simulink model "PRO_TestHarness"  (Simulink 8.6)
settings: Solver=ode45  StartTime=0.0  StopTime=10.0  RelTol=1e-3
PreLoadFcn:
  | addpath('./Workspace/')
  | load('./Workspace/EnvVar.mat')
  | if exist('tl_preloadfcn','file'), tl_preloadfcn(gcs,402); end
PostLoadFcn:
  | if exist('tl_postloadfcn','file'), tl_postloadfcn(gcs,402); end
InitFcn:
  | if exist('tlds_init','file'), tlds_init(gcs); end
StartFcn:
  | if exist('tlds_start','file'), tlds_start(gcs); end
StopFcn:
  | if exist('tlds_stop','file'), tlds_stop(gcs); end
undefined symbols (not defined in the file or in its folder): ddv, sigbuilder_block, Ts
libraries: tllib x19, simulink x2
(part 2 of 5)

== system PRO_TestHarness/PRO_AC_ProductionCycles/Subsystem/PRO_AC_ProductionCycles/PRO_AC_ProductionCycles/PRO_runProductionCycles ==
  u8RequestedCycle : Inport  OutDataTypeStr=uint8  PortDimensions=1  mask(TL_Inport){data={'autosar',{'useautosarcommunication',1,'kind',4,'senderreceiverport','prrDiagRequestCycle','dataelement','u8RequestedCycle','interrunnablevariable','BPA_AC_BeltParkingAlgorithm/IRV/u8BeltParkingAuthorizationState','clientserverport','pclDiagRequestCycle','operation','GetDiagRequestCycle'},'date',736040.52059280092}}
      settings: CopyFcn=if exist('tl_reset_reviewflag','file')==2,tl_reset_reviewflag(gcbh);end  DeleteFcn=if exist('delete_tlblock','file')==2,delete_tlblock(gcbh);end  NameChangeFcn=if exist('rename_tlblock','file')==2,rename_tlblock(gcbh);end  OpenFcn=if exist('tl_open_blockdlg','file')==2,tl_open_blockdlg(gcbh);else,open_system(gcbh,'parameter');end
      mask Help: eval(['if exist(''tl_online_help'',''file'') == 2, tl_online_help(''Topic'',''TL_Inport''),else, web([''jar:file:///'',matlabroot,''/help/toolbox/simulink/help.jar!/slref/' lower(get_param(gcbh,'Blocktype')) '.html''], ''-helpbrowser''),end'])
      mask Display: plot([0.2 0.35 NaN 0.65 0.8],[0 1 NaN 0 1]);
  u8ExecutedCycle : Inport  Port=2  PortDimensions=1  mask(TL_Inport){data={'autosar',{'useautosarcommunication',1,'senderreceiverport','prrExecutedCycle','dataelement','u8CycleNumber'},'date',735609.60262215277}}
      settings: CopyFcn=if exist('tl_reset_reviewflag','file')==2,tl_reset_reviewflag(gcbh);end  DeleteFcn=if exist('delete_tlblock','file')==2,delete_tlblock(gcbh);end  NameChangeFcn=if exist('rename_tlblock','file')==2,rename_tlblock(gcbh);end  OpenFcn=if exist('tl_open_blockdlg','file')==2,tl_open_blockdlg(gcbh);else,open_system(gcbh,'parameter');end
      mask Help: eval(['if exist(''tl_online_help'',''file'') == 2, tl_online_help(''Topic'',''TL_Inport''),else, web([''jar:file:///'',matlabroot,''/help/toolbox/simulink/help.jar!/slref/' lower(get_param(gcbh,'Blocktype')) '.html''], ''-helpbrowser''),end'])
      mask Display: plot([0.2 0.35 NaN 0.65 0.8],[0 1 NaN 0 1]);
  Trigger : TriggerPort  RequirementInfo={} %GIDa_248c7611_0acb_4b44_ba04_7ddf45d8e22c  TriggerType=function-call
  Constant2 : Constant  Value=ddv('BFD/CFG_K_MASK_PRO_DTC_ABORTION_CONTEXT')  OutDataTypeStr=uint8  mask(TL_Constant){data={'output',{'variable','BFD/CFG_K_MASK_PRO_DTC_ABORTION_CONTEXT'},'date',735893.56781245372}}
      settings: DeleteFcn=if exist('delete_tlblock','file')==2,delete_tlblock(gcbh);end  NameChangeFcn=if exist('rename_tlblock','file')==2,rename_tlblock(gcbh);end  OpenFcn=if exist('tl_open_blockdlg','file')==2,tl_open_blockdlg(gcbh);else,open_system(gcbh,'parameter');end
      mask Help: eval(['if exist(''tl_online_help'',''file'') == 2, tl_online_help(''Topic'',''TL_Constant''),else, web([''jar:file:///'',matlabroot,''/help/toolbox/simulink/help.jar!/slref/' lower(get_param(gcbh,'Blocktype')) '.html''], ''-helpbrowser''),end'])
      mask Display: plot([-0.05, 1.05, NaN, -0.05, 1.05],[.01, .01, NaN, .99, .99])
  Constant4 : Constant  Value=ddv('BFD/CFG_K_MASK_PRO_DTC_INHIBITION_CONTEXT')  OutDataTypeStr=uint8  mask(TL_Constant){data={'output',{'variable','BFD/CFG_K_MASK_PRO_DTC_INHIBITION_CONTEXT'},'date',735893.56753854163}}
      settings: DeleteFcn=if exist('delete_tlblock','file')==2,delete_tlblock(gcbh);end  NameChangeFcn=if exist('rename_tlblock','file')==2,rename_tlblock(gcbh);end  OpenFcn=if exist('tl_open_blockdlg','file')==2,tl_open_blockdlg(gcbh);else,open_system(gcbh,'parameter');end
      mask Help: eval(['if exist(''tl_online_help'',''file'') == 2, tl_online_help(''Topic'',''TL_Constant''),else, web([''jar:file:///'',matlabroot,''/help/toolbox/simulink/help.jar!/slref/' lower(get_param(gcbh,'Blocktype')) '.html''], ''-helpbrowser''),end'])
      mask Display: plot([-0.05, 1.05, NaN, -0.05, 1.05],[.01, .01, NaN, .99, .99])
  Dem_GetEventStatus : Subsystem  RequirementInfo={} %GIDa_e11a4632_883c_4bf9_94c9_e29d5c312dd8  TreatAsAtomicUnit=on
  Dem_GetEventStatus1 : Subsystem  RequirementInfo={} %GIDa_4470c0a2_043c_4322_94f3_9034f61d5407  TreatAsAtomicUnit=on
  Flags_PRO1 : Subsystem
  Flags_PRO2 : Subsystem
  PRO enabled : Subsystem  TreatAsAtomicUnit=on
  Runnable : tllib/Function  data={'autosar',{'useautosarspecification',1,'softwarecomponent','AUTOLIV/SoftwareComponents/PRO/PRO_AC_ProductionCycles','runnable','PRO_runProductionCycles'},'date',736811.32660734956}  displayString=RUNNABLE
  SCA_runCheckSystemContext1 : Subsystem  RequirementInfo={} %GIDa_959a77de_17ea_490b_b4e4_7bbcc1f3502a  TreatAsAtomicUnit=on
  SCA_runCheckSystemContext2 : Subsystem  RequirementInfo={} %GIDa_6e6b4e65_c2e0_44f1_91eb_aa27d502d2da  TreatAsAtomicUnit=on
  b8TriggeringOrder_PRO1 : Outport  PortDimensions=1  mask(TL_Outport){data={'autosar',{'useautosarcommunication',1,'senderreceiverport','psrAlgo_Flags_PRO1','dataelement','b8TriggerFlag'},'date',735664.44418690971}}
      settings: CopyFcn=if exist('tl_reset_reviewflag','file')==2,tl_reset_reviewflag(gcbh);end  DeleteFcn=if exist('delete_tlblock','file')==2,delete_tlblock(gcbh);end  NameChangeFcn=if exist('rename_tlblock','file')==2,rename_tlblock(gcbh);end  OpenFcn=if exist('tl_open_blockdlg','file')==2,tl_open_blockdlg(gcbh);else,open_system(gcbh,'parameter');end
      mask Help: eval(['if exist(''tl_online_help'',''file'') == 2, tl_online_help(''Topic'',''TL_Outport''),else, web([''jar:file:///'',matlabroot,''/help/toolbox/simulink/help.jar!/slref/' lower(get_param(gcbh,'Blocktype')) '.html''], ''-helpbrowser''),end'])
      mask Display: plot([0.2 0.35 NaN 0.65 0.8],[0 1 NaN 0 1]);
  b8AbortionOrder_PRO1 : Outport  Port=2  PortDimensions=1  mask(TL_Outport){data={'autosar',{'useautosarcommunication',1,'senderreceiverport','psrAlgo_Flags_PRO1','dataelement','b8InterruptFlag'},'date',735664.44679810188}}
      settings: CopyFcn=if exist('tl_reset_reviewflag','file')==2,tl_reset_reviewflag(gcbh);end  DeleteFcn=if exist('delete_tlblock','file')==2,delete_tlblock(gcbh);end  NameChangeFcn=if exist('rename_tlblock','file')==2,rename_tlblock(gcbh);end  OpenFcn=if exist('tl_open_blockdlg','file')==2,tl_open_blockdlg(gcbh);else,open_system(gcbh,'parameter');end
      mask Help: eval(['if exist(''tl_online_help'',''file'') == 2, tl_online_help(''Topic'',''TL_Outport''),else, web([''jar:file:///'',matlabroot,''/help/toolbox/simulink/help.jar!/slref/' lower(get_param(gcbh,'Blocktype')) '.html''], ''-helpbrowser''),end'])
      mask Display: plot([0.2 0.35 NaN 0.65 0.8],[0 1 NaN 0 1]);
  b8PreActivationFlag_PRO1 : Outport  Port=3  PortDimensions=1  mask(TL_Outport){data={'autosar',{'useautosarcommunication',1,'senderreceiverport','psrAlgo_Flags_PRO1','dataelement','b8PreActivationFlag'},'date',735664.44689250004}}
      settings: CopyFcn=if exist('tl_reset_reviewflag','file')==2,tl_reset_reviewflag(gcbh);end  DeleteFcn=if exist('delete_tlblock','file')==2,delete_tlblock(gcbh);end  NameChangeFcn=if exist('rename_tlblock','file')==2,rename_tlblock(gcbh);end  OpenFcn=if exist('tl_open_blockdlg','file')==2,tl_open_blockdlg(gcbh);else,open_system(gcbh,'parameter');end
      mask Help: eval(['if exist(''tl_online_help'',''file'') == 2, tl_online_help(''Topic'',''TL_Outport''),else, web([''jar:file:///'',matlabroot,''/help/toolbox/simulink/help.jar!/slref/' lower(get_param(gcbh,'Blocktype')) '.html''], ''-helpbrowser''),end'])
      mask Display: plot([0.2 0.35 NaN 0.65 0.8],[0 1 NaN 0 1]);
  b8PreConditionsFlag_PRO1 : Outport  Port=4  PortDimensions=1  mask(TL_Outport){data={'autosar',{'useautosarcommunication',1,'senderreceiverport','psrAlgo_Flags_PRO1','dataelement','b8PreConditionsFlag'},'date',735664.44697152777}}
      settings: CopyFcn=if exist('tl_reset_reviewflag','file')==2,tl_reset_reviewflag(gcbh);end  DeleteFcn=if exist('delete_tlblock','file')==2,delete_tlblock(gcbh);end  NameChangeFcn=if exist('rename_tlblock','file')==2,rename_tlblock(gcbh);end  OpenFcn=if exist('tl_open_blockdlg','file')==2,tl_open_blockdlg(gcbh);else,open_system(gcbh,'parameter');end
      mask Help: eval(['if exist(''tl_online_help'',''file'') == 2, tl_online_help(''Topic'',''TL_Outport''),else, web([''jar:file:///'',matlabroot,''/help/toolbox/simulink/help.jar!/slref/' lower(get_param(gcbh,'Blocktype')) '.html''], ''-helpbrowser''),end'])
      mask Display: plot([0.2 0.35 NaN 0.65 0.8],[0 1 NaN 0 1]);
  u8TriggeringSource_PRO1 : Outport  Port=5  PortDimensions=1  mask(TL_Outport){data={'autosar',{'useautosarcommunication',1,'senderreceiverport','psrAlgo_Flags_PRO1','dataelement','u8TriggeringSource'},'date',735664.44705670141}}
      settings: CopyFcn=if exist('tl_reset_reviewflag','file')==2,tl_reset_reviewflag(gcbh);end  DeleteFcn=if exist('delete_tlblock','file')==2,delete_tlblock(gcbh);end  NameChangeFcn=if exist('rename_tlblock','file')==2,rename_tlblock(gcbh);end  OpenFcn=if exist('tl_open_blockdlg','file')==2,tl_open_blockdlg(gcbh);else,open_system(gcbh,'parameter');end
      mask Help: eval(['if exist(''tl_online_help'',''file'') == 2, tl_online_help(''Topic'',''TL_Outport''),else, web([''jar:file:///'',matlabroot,''/help/toolbox/simulink/help.jar!/slref/' lower(get_param(gcbh,'Blocktype')) '.html''], ''-helpbrowser''),end'])
      mask Display: plot([0.2 0.35 NaN 0.65 0.8],[0 1 NaN 0 1]);
  b8TriggeringOrder_PRO2 : Outport  Port=6  PortDimensions=1  mask(TL_Outport){data={'autosar',{'useautosarcommunication',1,'senderreceiverport','psrAlgo_Flags_PRO2','dataelement','b8TriggerFlag'},'date',735664.44714405097}}
      settings: CopyFcn=if exist('tl_reset_reviewflag','file')==2,tl_reset_reviewflag(gcbh);end  DeleteFcn=if exist('delete_tlblock','file')==2,delete_tlblock(gcbh);end  NameChangeFcn=if exist('rename_tlblock','file')==2,rename_tlblock(gcbh);end  OpenFcn=if exist('tl_open_blockdlg','file')==2,tl_open_blockdlg(gcbh);else,open_system(gcbh,'parameter');end
      mask Help: eval(['if exist(''tl_online_help'',''file'') == 2, tl_online_help(''Topic'',''TL_Outport''),else, web([''jar:file:///'',matlabroot,''/help/toolbox/simulink/help.jar!/slref/' lower(get_param(gcbh,'Blocktype')) '.html''], ''-helpbrowser''),end'])
      mask Display: plot([0.2 0.35 NaN 0.65 0.8],[0 1 NaN 0 1]);
  b8AbortionOrder_PRO2 : Outport  Port=7  PortDimensions=1  mask(TL_Outport){data={'autosar',{'useautosarcommunication',1,'senderreceiverport','psrAlgo_Flags_PRO2','dataelement','b8InterruptFlag'},'date',735664.44722253468}}
      settings: CopyFcn=if exist('tl_reset_reviewflag','file')==2,tl_reset_reviewflag(gcbh);end  DeleteFcn=if exist('delete_tlblock','file')==2,delete_tlblock(gcbh);end  NameChangeFcn=if exist('rename_tlblock','file')==2,rename_tlblock(gcbh);end  OpenFcn=if exist('tl_open_blockdlg','file')==2,tl_open_blockdlg(gcbh);else,open_system(gcbh,'parameter');end
      mask Help: eval(['if exist(''tl_online_help'',''file'') == 2, tl_online_help(''Topic'',''TL_Outport''),else, web([''jar:file:///'',matlabroot,''/help/toolbox/simulink/help.jar!/slref/' lower(get_param(gcbh,'Blocktype')) '.html''], ''-helpbrowser''),end'])
      mask Display: plot([0.2 0.35 NaN 0.65 0.8],[0 1 NaN 0 1]);
  b8PreActivationFlag_PRO2 : Outport  Port=8  PortDimensions=1  mask(TL_Outport){data={'autosar',{'useautosarcommunication',1,'senderreceiverport','psrAlgo_Flags_PRO2','dataelement','b8PreActivationFlag'},'date',735664.44730300922}}
      settings: CopyFcn=if exist('tl_reset_reviewflag','file')==2,tl_reset_reviewflag(gcbh);end  DeleteFcn=if exist('delete_tlblock','file')==2,delete_tlblock(gcbh);end  NameChangeFcn=if exist('rename_tlblock','file')==2,rename_tlblock(gcbh);end  OpenFcn=if exist('tl_open_blockdlg','file')==2,tl_open_blockdlg(gcbh);else,open_system(gcbh,'parameter');end
      mask Help: eval(['if exist(''tl_online_help'',''file'') == 2, tl_online_help(''Topic'',''TL_Outport''),else, web([''jar:file:///'',matlabroot,''/help/toolbox/simulink/help.jar!/slref/' lower(get_param(gcbh,'Blocktype')) '.html''], ''-helpbrowser''),end'])
      mask Display: plot([0.2 0.35 NaN 0.65 0.8],[0 1 NaN 0 1]);
  b8PreConditionsFlag_PRO2 : Outport  Port=9  PortDimensions=1  mask(TL_Outport){data={'autosar',{'useautosarcommunication',1,'senderreceiverport','psrAlgo_Flags_PRO2','dataelement','b8PreConditionsFlag'},'date',735664.44739415508}}
      settings: CopyFcn=if exist('tl_reset_reviewflag','file')==2,tl_reset_reviewflag(gcbh);end  DeleteFcn=if exist('delete_tlblock','file')==2,delete_tlblock(gcbh);end  NameChangeFcn=if exist('rename_tlblock','file')==2,rename_tlblock(gcbh);end  OpenFcn=if exist('tl_open_blockdlg','file')==2,tl_open_blockdlg(gcbh);else,open_system(gcbh,'parameter');end
      mask Help: eval(['if exist(''tl_online_help'',''file'') == 2, tl_online_help(''Topic'',''TL_Outport''),else, web([''jar:file:///'',matlabroot,''/help/toolbox/simulink/help.jar!/slref/' lower(get_param(gcbh,'Blocktype')) '.html''], ''-helpbrowser''),end'])
      mask Display: plot([0.2 0.35 NaN 0.65 0.8],[0 1 NaN 0 1]);
  u8TriggeringSource_PRO2 : Outport  Port=10  PortDimensions=1  mask(TL_Outport){data={'autosar',{'useautosarcommunication',1,'senderreceiverport','psrAlgo_Flags_PRO2','dataelement','u8TriggeringSource'},'date',735664.44747879624}}
      settings: CopyFcn=if exist('tl_reset_reviewflag','file')==2,tl_reset_reviewflag(gcbh);end  DeleteFcn=if exist('delete_tlblock','file')==2,delete_tlblock(gcbh);end  NameChangeFcn=if exist('rename_tlblock','file')==2,rename_tlblock(gcbh);end  OpenFcn=if exist('tl_open_blockdlg','file')==2,tl_open_blockdlg(gcbh);else,open_system(gcbh,'parameter');end
      mask Help: eval(['if exist(''tl_online_help'',''file'') == 2, tl_online_help(''Topic'',''TL_Outport''),else, web([''jar:file:///'',matlabroot,''/help/toolbox/simulink/help.jar!/slref/' lower(get_param(gcbh,'Blocktype')) '.html''], ''-helpbrowser''),end'])
      mask Display: plot([0.2 0.35 NaN 0.65 0.8],[0 1 NaN 0 1]);
  wires:
  u8ExecutedCycle/1 -> PRO enabled/2(u8ExecutedCycle)
  SCA_runCheckSystemContext1/1(b8SystemContext) -> PRO enabled/3(b8SystemContextInhibition)
  SCA_runCheckSystemContext2/1(b8SystemContext) -> PRO enabled/4(b8SystemContextAbortion)
  Constant2/1 -> SCA_runCheckSystemContext2/1(u16SystemContextsToCheck)
  u8RequestedCycle/1 -> PRO enabled/1(u8RequestedCycle)
  Constant4/1 -> SCA_runCheckSystemContext1/1(u16SystemContextsToCheck)
  PRO enabled/1(psrAlgoFlags_PRO1) -> Flags_PRO1/1(In1)
  Flags_PRO1/1(Out1) -> b8TriggeringOrder_PRO1/1
  Flags_PRO1/2(Out2) -> b8AbortionOrder_PRO1/1
  Flags_PRO1/3(Out3) -> b8PreActivationFlag_PRO1/1
  Flags_PRO1/4(Out4) -> b8PreConditionsFlag_PRO1/1
  Flags_PRO1/5(Out5) -> u8TriggeringSource_PRO1/1
  Flags_PRO2/1(Out1) -> b8TriggeringOrder_PRO2/1
  Flags_PRO2/2(Out2) -> b8AbortionOrder_PRO2/1
  Flags_PRO2/3(Out3) -> b8PreActivationFlag_PRO2/1
  Flags_PRO2/4(Out4) -> b8PreConditionsFlag_PRO2/1
  Flags_PRO2/5(Out5) -> u8TriggeringSource_PRO2/1
  PRO enabled/2(psrAlgoFlags_PRO2) -> Flags_PRO2/1(In1)
  Dem_GetEventStatus1/1(u8EventStatus) -> PRO enabled/5(u8UVDuringTensioningEventStatus)
  Dem_GetEventStatus/1(u8EventStatus) -> PRO enabled/6(u8OverVoltageEventStatus)

== system PRO_TestHarness/PRO_AC_ProductionCycles/Subsystem/PRO_AC_ProductionCycles/PRO_AC_ProductionCycles/WriteSystemContextOutputs ==
  b8CyclesInhibitedByDTC1 : Inport
  b8CyclesAbortedByDTC : Inport  Port=2
  u8AecStatus_UVDuringTens1 : Inport  Port=3
  u8Status_OVO : Inport  Port=4
  Trigger : TriggerPort  RequirementInfo={} %GIDa_0b5c07fd_5561_4776_a0f4_36f279c5ca10  TriggerType=function-call
  Data Store Write1 : DataStoreWrite  DataStoreName=b8CyclesInhibitedByDTC  mask(TL_DataStoreWrite){data={'date',735893.56874431716}}
      settings: DeleteFcn=if exist('delete_tlblock','file')==2,delete_tlblock(gcbh);end  NameChangeFcn=if exist('rename_tlblock','file')==2,rename_tlblock(gcbh);end  OpenFcn=if exist('tl_open_blockdlg','file')==2,tl_open_blockdlg(gcbh);else,open_system(gcbh,'parameter');end
      mask Help: eval(['if exist(''tl_online_help'',''file'') == 2, tl_online_help(''Topic'',''TL_DataStoreWrite''),else, web([''jar:file:///'',matlabroot,''/help/toolbox/simulink/help.jar!/slref/' lower(get_param(gcbh,'Blocktype')) '.html''], ''-helpbrowser''),end'])
      mask Display: plot([-0.05, 1.05, NaN, -0.05, 1.05],[.01, .01, NaN, .99, .99])
  Data Store Write2 : DataStoreWrite  DataStoreName=b8CyclesAbortedByDTC  mask(TL_DataStoreWrite){data={'date',735893.56880297454}}
      settings: DeleteFcn=if exist('delete_tlblock','file')==2,delete_tlblock(gcbh);end  NameChangeFcn=if exist('rename_tlblock','file')==2,rename_tlblock(gcbh);end  OpenFcn=if exist('tl_open_blockdlg','file')==2,tl_open_blockdlg(gcbh);else,open_system(gcbh,'parameter');end
      mask Help: eval(['if exist(''tl_online_help'',''file'') == 2, tl_online_help(''Topic'',''TL_DataStoreWrite''),else, web([''jar:file:///'',matlabroot,''/help/toolbox/simulink/help.jar!/slref/' lower(get_param(gcbh,'Blocktype')) '.html''], ''-helpbrowser''),end'])
      mask Display: plot([-0.05, 1.05, NaN, -0.05, 1.05],[.01, .01, NaN, .99, .99])
  Data Store Write4 : DataStoreWrite  DataStoreName=u8Status_UVT  mask(TL_DataStoreWrite){data={'date',736231.39905967598}}
      settings: DeleteFcn=if exist('delete_tlblock','file')==2,delete_tlblock(gcbh);end  NameChangeFcn=if exist('rename_tlblock','file')==2,rename_tlblock(gcbh);end  OpenFcn=if exist('tl_open_blockdlg','file')==2,tl_open_blockdlg(gcbh);else,open_system(gcbh,'parameter');end
      mask Help: eval(['if exist(''tl_online_help'',''file'') == 2, tl_online_help(''Topic'',''TL_DataStoreWrite''),else, web([''jar:file:///'',matlabroot,''/help/toolbox/simulink/help.jar!/slref/' lower(get_param(gcbh,'Blocktype')) '.html''], ''-helpbrowser''),end'])
      mask Display: plot([-0.05, 1.05, NaN, -0.05, 1.05],[.01, .01, NaN, .99, .99])
  Data Store Write5 : DataStoreWrite  DataStoreName=u8Status_OVO  mask(TL_DataStoreWrite){data={'date',735987.71420101856}}
      settings: DeleteFcn=if exist('delete_tlblock','file')==2,delete_tlblock(gcbh);end  NameChangeFcn=if exist('rename_tlblock','file')==2,rename_tlblock(gcbh);end  OpenFcn=if exist('tl_open_blockdlg','file')==2,tl_open_blockdlg(gcbh);else,open_system(gcbh,'parameter');end
      mask Help: eval(['if exist(''tl_online_help'',''file'') == 2, tl_online_help(''Topic'',''TL_DataStoreWrite''),else, web([''jar:file:///'',matlabroot,''/help/toolbox/simulink/help.jar!/slref/' lower(get_param(gcbh,'Blocktype')) '.html''], ''-helpbrowser''),end'])
      mask Display: plot([-0.05, 1.05, NaN, -0.05, 1.05],[.01, .01, NaN, .99, .99])
  wires:
  b8CyclesInhibitedByDTC1/1 -> Data Store Write1/1
  b8CyclesAbortedByDTC/1 -> Data Store Write2/1
  u8AecStatus_UVDuringTens1/1 -> Data Store Write4/1
  u8Status_OVO/1 -> Data Store Write5/1

== system PRO_TestHarness/PRO_AC_ProductionCycles/Subsystem/PRO_AC_ProductionCycles/PRO_AC_ProductionCycles/PRO_runProductionCycles/Dem_GetEventStatus ==
  Data Store Read1 : DataStoreRead  DataStoreName=u8Status_OVO  mask(TL_DataStoreRead){data={'date',735987.66306642361}}
      settings: DeleteFcn=if exist('delete_tlblock','file')==2,delete_tlblock(gcbh);end  NameChangeFcn=if exist('rename_tlblock','file')==2,rename_tlblock(gcbh);end  OpenFcn=if exist('tl_open_blockdlg','file')==2,tl_open_blockdlg(gcbh);else,open_system(gcbh,'parameter');end
      mask Help: eval(['if exist(''tl_online_help'',''file'') == 2, tl_online_help(''Topic'',''TL_DataStoreRead''),else, web([''jar:file:///'',matlabroot,''/help/toolbox/simulink/help.jar!/slref/' lower(get_param(gcbh,'Blocktype')) '.html''], ''-helpbrowser''),end'])
      mask Display: plot([-0.05, 1.05, NaN, -0.05, 1.05],[.01, .01, NaN, .99, .99])
  Function1 : tllib/Function  RequirementInfo={} %GIDa_c22adf50_ccfc_4787_ab66_0286f94d3b05  data={'stepfunctionname','Rte_Call_pclSystemContext_CheckSystemContext','stepfunctionclass','EXTERN_FCN_SCA','functionarglist',{'u16SystemContextsToCheck';'b8SystemContextStatus_DTCInhibition'},'autosar',{'useautosarspecification',1,'functionrole',3,'clientport','pclEvtInfoBatPwrOverVoltage','operation','GetEventStatus','isimplementationforsilpil',0,'clientsoftwarecomponent','AUTOLIV/SoftwareComponents/PRO/PRO_AC_ProductionCycles'},'date',736811.33406144672}  displayString=|
      | OPERATION CALL
      | (SYNCHRONOUS)
  u8EventStatus : Outport  RequirementInfo={} %GIDa_cf1b259b_4028_4359_97b1_6f9420fe6927  PortDimensions=1  mask(TL_Outport){data={'output',{'name','$B','max',255,'min',0,'class','FCN_REF_ARG','type','UInt8'},'autosar',{'useautosarcommunication',1,'kind',5,'operationargument','AUTOSAR_Dem/ASR42/PortInterfaces/Dem_ASR42_DiagnosticInfo/Operations/GetEventStatus/OperationArguments/EventStatusExtended'},'date',736811.33321328706}}
      settings: CopyFcn=if exist('tl_reset_reviewflag','file')==2,tl_reset_reviewflag(gcbh);end  DeleteFcn=if exist('delete_tlblock','file')==2,delete_tlblock(gcbh);end  NameChangeFcn=if exist('rename_tlblock','file')==2,rename_tlblock(gcbh);end  OpenFcn=if exist('tl_open_blockdlg','file')==2,tl_open_blockdlg(gcbh);else,open_system(gcbh,'parameter');end
      mask Help: eval(['if exist(''tl_online_help'',''file'') == 2, tl_online_help(''Topic'',''TL_Outport''),else, web([''jar:file:///'',matlabroot,''/help/toolbox/simulink/help.jar!/slref/' lower(get_param(gcbh,'Blocktype')) '.html''], ''-helpbrowser''),end'])
      mask Display: plot([0.2 0.35 NaN 0.65 0.8],[0 1 NaN 0 1]);
  u8OperationStatus : Outport  RequirementInfo={} %GIDa_4a7fdf99_1c8f_4d14_82e9_ce5d358773f6  Port=2  PortDimensions=1  mask(TL_Outport){data={'output',{'name','$B','max',255,'min',0,'class','FCN_REF_ARG','type','UInt8'},'autosar',{'useautosarcommunication',1,'kind',6,'operationargument','AUTOSAR_Dem/ASR42/PortInterfaces/Dem_ASR42_DiagnosticInfo/Operations/GetEventStatus/OperationArguments/EventStatusExtended'},'date',736811.33358806709}}
      settings: CopyFcn=if exist('tl_reset_reviewflag','file')==2,tl_reset_reviewflag(gcbh);end  DeleteFcn=if exist('delete_tlblock','file')==2,delete_tlblock(gcbh);end  NameChangeFcn=if exist('rename_tlblock','file')==2,rename_tlblock(gcbh);end  OpenFcn=if exist('tl_open_blockdlg','file')==2,tl_open_blockdlg(gcbh);else,open_system(gcbh,'parameter');end
      mask Help: eval(['if exist(''tl_online_help'',''file'') == 2, tl_online_help(''Topic'',''TL_Outport''),else, web([''jar:file:///'',matlabroot,''/help/toolbox/simulink/help.jar!/slref/' lower(get_param(gcbh,'Blocktype')) '.html''], ''-helpbrowser''),end'])
      mask Display: plot([0.2 0.35 NaN 0.65 0.8],[0 1 NaN 0 1]);
  wires:
  Data Store Read1/1 -> u8EventStatus/1

== system PRO_TestHarness/PRO_AC_ProductionCycles/Subsystem/PRO_AC_ProductionCycles/PRO_AC_ProductionCycles/PRO_runProductionCycles/Dem_GetEventStatus1 ==
  Data Store Read2 : DataStoreRead  DataStoreName=u8Status_UVT  mask(TL_DataStoreRead){data={'date',736231.39714105322}}
      settings: DeleteFcn=if exist('delete_tlblock','file')==2,delete_tlblock(gcbh);end  NameChangeFcn=if exist('rename_tlblock','file')==2,rename_tlblock(gcbh);end  OpenFcn=if exist('tl_open_blockdlg','file')==2,tl_open_blockdlg(gcbh);else,open_system(gcbh,'parameter');end
      mask Help: eval(['if exist(''tl_online_help'',''file'') == 2, tl_online_help(''Topic'',''TL_DataStoreRead''),else, web([''jar:file:///'',matlabroot,''/help/toolbox/simulink/help.jar!/slref/' lower(get_param(gcbh,'Blocktype')) '.html''], ''-helpbrowser''),end'])
      mask Display: plot([-0.05, 1.05, NaN, -0.05, 1.05],[.01, .01, NaN, .99, .99])
  Function : tllib/Function  RequirementInfo={} %GIDa_f447fc35_00c3_4c09_bd92_7698dee7f982  data={'stepfunctionname','Rte_Call_pclSystemContext_CheckSystemContext','stepfunctionclass','EXTERN_FCN_SCA','functionarglist',{'u16SystemContextsToCheck';'b8SystemContextStatus_DTCInhibition'},'autosar',{'useautosarspecification',1,'functionrole',3,'clientport','pclEvtInfoBatPwrUnderVoltageDuringTens','operation','GetEventStatus','isimplementationforsilpil',0,'clientsoftwarecomponent','AUTOLIV/SoftwareComponents/PRO/PRO_AC_ProductionCycles'},'date',736811.33328623837}  displayString=|
      | OPERATION CALL
      | (SYNCHRONOUS)
  u8EventStatus : Outport  RequirementInfo={} %GIDa_d61cb967_a741_4828_b426_163175ca575e  PortDimensions=1  mask(TL_Outport){data={'output',{'name','$B','max',255,'min',0,'class','FCN_REF_ARG','type','UInt8'},'autosar',{'useautosarcommunication',1,'kind',5,'operationargument','AUTOSAR_Dem/ASR42/PortInterfaces/Dem_ASR42_DiagnosticInfo/Operations/GetEventStatus/OperationArguments/EventStatusExtended'},'date',736811.33321328706}}
      settings: CopyFcn=if exist('tl_reset_reviewflag','file')==2,tl_reset_reviewflag(gcbh);end  DeleteFcn=if exist('delete_tlblock','file')==2,delete_tlblock(gcbh);end  NameChangeFcn=if exist('rename_tlblock','file')==2,rename_tlblock(gcbh);end  OpenFcn=if exist('tl_open_blockdlg','file')==2,tl_open_blockdlg(gcbh);else,open_system(gcbh,'parameter');end
      mask Help: eval(['if exist(''tl_online_help'',''file'') == 2, tl_online_help(''Topic'',''TL_Outport''),else, web([''jar:file:///'',matlabroot,''/help/toolbox/simulink/help.jar!/slref/' lower(get_param(gcbh,'Blocktype')) '.html''], ''-helpbrowser''),end'])
      mask Display: plot([0.2 0.35 NaN 0.65 0.8],[0 1 NaN 0 1]);
  u8OperationStatus : Outport  RequirementInfo={} %GIDa_0497bde6_0e2f_4479_a6c2_fbaaba97d3b8  Port=2  PortDimensions=1  mask(TL_Outport){data={'output',{'name','$B','max',255,'min',0,'class','FCN_REF_ARG','type','UInt8'},'autosar',{'useautosarcommunication',1,'kind',6,'operationargument','AUTOSAR_Dem/ASR42/PortInterfaces/Dem_ASR42_DiagnosticInfo/Operations/GetEventStatus/OperationArguments/EventStatusExtended'},'date',736811.33358806709}}
      settings: CopyFcn=if exist('tl_reset_reviewflag','file')==2,tl_reset_reviewflag(gcbh);end  DeleteFcn=if exist('delete_tlblock','file')==2,delete_tlblock(gcbh);end  NameChangeFcn=if exist('rename_tlblock','file')==2,rename_tlblock(gcbh);end  OpenFcn=if exist('tl_open_blockdlg','file')==2,tl_open_blockdlg(gcbh);else,open_system(gcbh,'parameter');end
      mask Help: eval(['if exist(''tl_online_help'',''file'') == 2, tl_online_help(''Topic'',''TL_Outport''),else, web([''jar:file:///'',matlabroot,''/help/toolbox/simulink/help.jar!/slref/' lower(get_param(gcbh,'Blocktype')) '.html''], ''-helpbrowser''),end'])
      mask Display: plot([0.2 0.35 NaN 0.65 0.8],[0 1 NaN 0 1]);
  wires:
  Data Store Read2/1 -> u8EventStatus/1

== system PRO_TestHarness/PRO_AC_ProductionCycles/Subsystem/PRO_AC_ProductionCycles/PRO_AC_ProductionCycles/PRO_runProductionCycles/Flags_PRO1 ==
  In1 : Inport
  BusSelector6 : BusSelector  OutputSignals=b8TriggerFlag_PRO,b8InterruptFlag_PRO,b8PreActivationFlag_PRO,b8PreConditionsFlag_PRO,u8TriggeringSource_PRO
  Out1 : Outport
  Out2 : Outport  Port=2
  Out3 : Outport  Port=3
  Out4 : Outport  Port=4
  Out5 : Outport  Port=5
  wires:
  In1/1 -> BusSelector6/1
  BusSelector6/1 -> Out1/1  "<b8TriggerFlag_PRO>"
  BusSelector6/2 -> Out2/1  "<b8InterruptFlag_PRO>"
  BusSelector6/3 -> Out3/1  "<b8PreActivationFlag_PRO>"
  BusSelector6/4 -> Out4/1  "<b8PreConditionsFlag_PRO>"
  BusSelector6/5 -> Out5/1  "<u8TriggeringSource_PRO>"

== system PRO_TestHarness/PRO_AC_ProductionCycles/Subsystem/PRO_AC_ProductionCycles/PRO_AC_ProductionCycles/PRO_runProductionCycles/Flags_PRO2 ==
  In1 : Inport
  BusSelector3 : BusSelector  OutputSignals=b8TriggerFlag_PRO,b8InterruptFlag_PRO,b8PreActivationFlag_PRO,b8PreConditionsFlag_PRO,u8TriggeringSource_PRO
  Out1 : Outport
  Out2 : Outport  Port=2
  Out3 : Outport  Port=3
  Out4 : Outport  Port=4
  Out5 : Outport  Port=5
  wires:
  In1/1 -> BusSelector3/1
  BusSelector3/2 -> Out2/1  "<b8InterruptFlag_PRO>"
  BusSelector3/4 -> Out4/1  "<b8PreConditionsFlag_PRO>"
  BusSelector3/5 -> Out5/1  "<u8TriggeringSource_PRO>"
  BusSelector3/1 -> Out1/1  "<b8TriggerFlag_PRO>"
  BusSelector3/3 -> Out3/1  "<b8PreActivationFlag_PRO>"

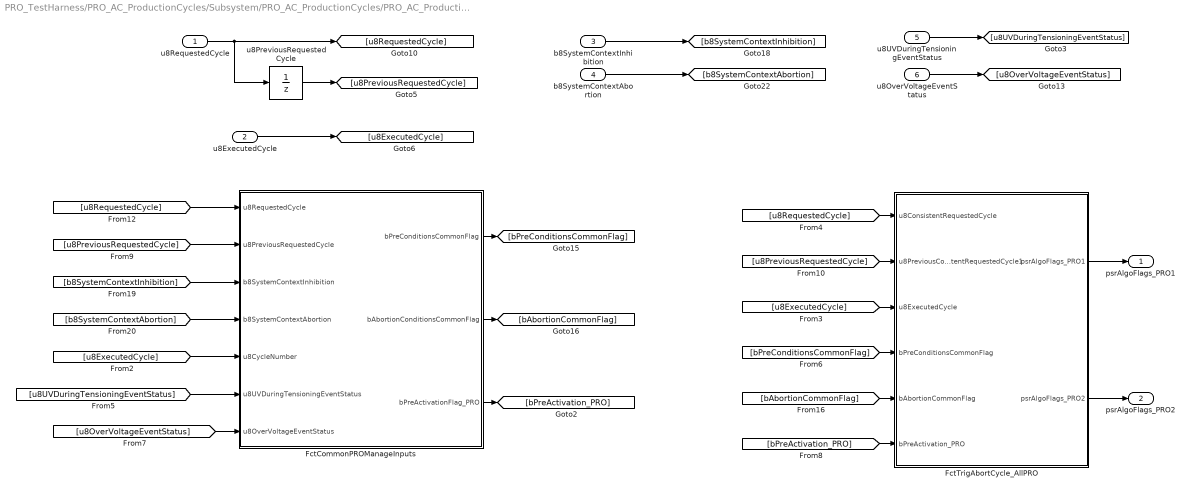
== system PRO_TestHarness/PRO_AC_ProductionCycles/Subsystem/PRO_AC_ProductionCycles/PRO_AC_ProductionCycles/PRO_runProductionCycles/PRO enabled ==
  u8RequestedCycle : Inport  OutDataTypeStr=uint8  PortDimensions=1
  u8ExecutedCycle : Inport  Port=2
  b8SystemContextInhibition : Inport  Port=3  OutDataTypeStr=uint8  PortDimensions=1
  b8SystemContextAbortion : Inport  Port=4  OutDataTypeStr=uint8  PortDimensions=1
  u8UVDuringTensioningEventStatus : Inport  Port=5
  u8OverVoltageEventStatus : Inport  Port=6
  FctCommonPROManageInputs : Subsystem  TreatAsAtomicUnit=on
  FctTrigAbortCycle_AllPRO : Subsystem  TreatAsAtomicUnit=on
  u8PreviousRequestedCycle : UnitDelay  InitialCondition=ddv('RTE_DEFINES/KU8_NO_CYCLE')  SampleTime=-1  mask(TL_UnitDelay){data={'output',{'name','$B','type','UInt8'},'state',{'name','X_$B','type','UInt8'},'date',736811.34437033569}}
      settings: CopyFcn=if exist('tl_reset_reviewflag') == 2, tl_reset_reviewflag(gcbh); end  DeleteFcn=if exist('delete_tlblock','file')==2,delete_tlblock(gcbh);end  NameChangeFcn=if exist('rename_tlblock','file')==2,rename_tlblock(gcbh);end  OpenFcn=if exist('tl_open_blockdlg','file')==2,tl_open_blockdlg(gcbh);else,open_system(gcbh,'parameter');end
      mask Help: eval(['if exist(''tl_online_help'',''file'') == 2, tl_online_help(''Topic'',''TL_UnitDelay''),else, web([''jar:file:///'',matlabroot,''/help/toolbox/simulink/help.jar!/slref/' lower(get_param(gcbh,'Blocktype')) '.html''], ''-helpbrowser''),end'])
      mask Display: plot([-0.05, 1.05, NaN, -0.05, 1.05],[.01, .01, NaN, .99, .99])
  psrAlgoFlags_PRO1 : Outport
  psrAlgoFlags_PRO2 : Outport  Port=2
  wires:
  u8ExecutedCycle/1 -> [u8ExecutedCycle]
  [u8ExecutedCycle] -> FctTrigAbortCycle_AllPRO/3(u8ExecutedCycle)
  b8SystemContextInhibition/1 -> [b8SystemContextInhibition]
  b8SystemContextAbortion/1 -> [b8SystemContextAbortion]
  u8RequestedCycle/1 -> u8PreviousRequestedCycle/1, [u8RequestedCycle]
  [u8RequestedCycle] -> FctCommonPROManageInputs/1(u8RequestedCycle)
  [u8RequestedCycle] -> FctTrigAbortCycle_AllPRO/1(u8ConsistentRequestedCycle)
  FctTrigAbortCycle_AllPRO/1(psrAlgoFlags_PRO1) -> psrAlgoFlags_PRO1/1
  FctCommonPROManageInputs/1(bPreConditionsCommonFlag) -> [bPreConditionsCommonFlag]
  FctCommonPROManageInputs/2(bAbortionConditionsCommonFlag) -> [bAbortionCommonFlag]
  [b8SystemContextAbortion] -> FctCommonPROManageInputs/4(b8SystemContextAbortion)
  [b8SystemContextInhibition] -> FctCommonPROManageInputs/3(b8SystemContextInhibition)
  [bPreConditionsCommonFlag] -> FctTrigAbortCycle_AllPRO/4(bPreConditionsCommonFlag)
  [bAbortionCommonFlag] -> FctTrigAbortCycle_AllPRO/5(bAbortionCommonFlag)
  FctTrigAbortCycle_AllPRO/2(psrAlgoFlags_PRO2) -> psrAlgoFlags_PRO2/1
  FctCommonPROManageInputs/3(bPreActivationFlag_PRO) -> [bPreActivation_PRO]
  [bPreActivation_PRO] -> FctTrigAbortCycle_AllPRO/6(bPreActivation_PRO)
  [u8ExecutedCycle] -> FctCommonPROManageInputs/5(u8CycleNumber)
  [u8PreviousRequestedCycle] -> FctTrigAbortCycle_AllPRO/2(u8PreviousConsistentRequestedCycle1)
  u8UVDuringTensioningEventStatus/1 -> [u8UVDuringTensioningEventStatus]
  [u8UVDuringTensioningEventStatus] -> FctCommonPROManageInputs/6(u8UVDuringTensioningEventStatus)
  u8OverVoltageEventStatus/1 -> [u8OverVoltageEventStatus]
  [u8OverVoltageEventStatus] -> FctCommonPROManageInputs/7(u8OverVoltageEventStatus)
  u8PreviousRequestedCycle/1 -> [u8PreviousRequestedCycle]
  [u8PreviousRequestedCycle] -> FctCommonPROManageInputs/2(u8PreviousRequestedCycle)

== system PRO_TestHarness/PRO_AC_ProductionCycles/Subsystem/PRO_AC_ProductionCycles/PRO_AC_ProductionCycles/PRO_runProductionCycles/SCA_runCheckSystemContext1 ==
  u16SystemContextsToCheck : Inport  PortDimensions=1  mask(TL_Inport){data={'output',{'class','FCN_ARG','type','UInt16'},'autosar',{'useautosarcommunication',1,'kind',5,'operationargument','AUTOLIV/GlobalDictionary/ClientServerInterfaces/icsModeManagement/Operations/CheckModeStatus/OperationArguments/u32ModesToCheck'},'date',736463.487601956}}
      settings: CopyFcn=if exist('tl_reset_reviewflag','file')==2,tl_reset_reviewflag(gcbh);end  DeleteFcn=if exist('delete_tlblock','file')==2,delete_tlblock(gcbh);end  NameChangeFcn=if exist('rename_tlblock','file')==2,rename_tlblock(gcbh);end  OpenFcn=if exist('tl_open_blockdlg','file')==2,tl_open_blockdlg(gcbh);else,open_system(gcbh,'parameter');end
      mask Help: eval(['if exist(''tl_online_help'',''file'') == 2, tl_online_help(''Topic'',''TL_Inport''),else, web([''jar:file:///'',matlabroot,''/help/toolbox/simulink/help.jar!/slref/' lower(get_param(gcbh,'Blocktype')) '.html''], ''-helpbrowser''),end'])
      mask Display: plot([0.2 0.35 NaN 0.65 0.8],[0 1 NaN 0 1]);
  Constant4 : Constant  Value=ddv('BFD/CFG_K_MASK_PRO_DTC_INHIBITION_CONTEXT')  OutDataTypeStr=uint8  mask(TL_Constant){data={'output',{'variable','BFD/CFG_K_MASK_PRO_DTC_INHIBITION_CONTEXT'},'date',735893.56754299765}}
      settings: DeleteFcn=if exist('delete_tlblock','file')==2,delete_tlblock(gcbh);end  NameChangeFcn=if exist('rename_tlblock','file')==2,rename_tlblock(gcbh);end  OpenFcn=if exist('tl_open_blockdlg','file')==2,tl_open_blockdlg(gcbh);else,open_system(gcbh,'parameter');end
      mask Help: eval(['if exist(''tl_online_help'',''file'') == 2, tl_online_help(''Topic'',''TL_Constant''),else, web([''jar:file:///'',matlabroot,''/help/toolbox/simulink/help.jar!/slref/' lower(get_param(gcbh,'Blocktype')) '.html''], ''-helpbrowser''),end'])
      mask Display: plot([-0.05, 1.05, NaN, -0.05, 1.05],[.01, .01, NaN, .99, .99])
  Function : tllib/Function  RequirementInfo={} %GIDa_c58da7a7_c804_42c4_9864_11873b795832  data={'stepfunctionname','Rte_Call_pclSystemContext_CheckSystemContext','stepfunctionclass','EXTERN_FCN_SCA','forcereuse',1,'functionarglist',{'u16SystemContextsToCheck';'b8SystemContextStatus_DTCInhibition'},'autosar',{'useautosarspecification',1,'functionrole',3,'clientport','pclModeManagement','operation','CheckModeStatus','isimplementationforsilpil',0,'clientsoftwarecomponent','AUTOLIV/SoftwareComponents/PRO/PRO_AC_ProductionCycles'},'date',736811.32660910883}  displayString=|
      | OPERATION CALL
      | (SYNCHRONOUS)
  If : If  IfExpression=u1
  If Action Subsystem1 : Subsystem  TreatAsAtomicUnit=on
  If Action Subsystem2 : Subsystem  TreatAsAtomicUnit=on
  Merge : Merge  InitialOutput=170  mask(TL_Merge){data={'date',735664.45352688653}}
      settings: CopyFcn=if exist('tl_reset_reviewflag') == 2, tl_reset_reviewflag(gcbh); end  DeleteFcn=if exist('delete_tlblock','file')==2,delete_tlblock(gcbh);end  NameChangeFcn=if exist('rename_tlblock','file')==2,rename_tlblock(gcbh);end  OpenFcn=if exist('tl_open_blockdlg','file')==2,tl_open_blockdlg(gcbh);else,open_system(gcbh,'parameter');end
      mask Help: eval(['if exist(''tl_online_help'',''file'') == 2, tl_online_help(''Topic'',''TL_Merge''),else, web([''jar:file:///'',matlabroot,''/help/toolbox/simulink/help.jar!/slref/' lower(get_param(gcbh,'Blocktype')) '.html''], ''-helpbrowser''),end'])
      mask Display: plot([-0.05, 1.05, NaN, -0.05, 1.05],[.01, .01, NaN, .99, .99])
  bNoInbibSystemCtxt : RelationalOperator  Operator===  OutDataTypeStr=boolean  mask(TL_RelationalOperator){data={'output',{'name','$B'},'date',735419.63408075226}}
      settings: DeleteFcn=if exist('delete_tlblock','file')==2,delete_tlblock(gcbh);end  NameChangeFcn=if exist('rename_tlblock','file')==2,rename_tlblock(gcbh);end  OpenFcn=if exist('tl_open_blockdlg','file')==2,tl_open_blockdlg(gcbh);else,open_system(gcbh,'parameter');end
      mask Help: eval(['if exist(''tl_online_help'',''file'') == 2, tl_online_help(''Topic'',''TL_RelationalOperator''),else, web([''jar:file:///'',matlabroot,''/help/toolbox/simulink/help.jar!/slref/' lower(get_param(gcbh,'Blocktype')) '.html''], ''-helpbrowser''),end'])
      mask Display: plot([-0.05, 1.05, NaN, -0.05, 1.05],[.01, .01, NaN, .99, .99])
  b8SystemContext : Outport  RequirementInfo={} %GIDa_df090813_2ed3_487a_91dc_abdc7380150a  PortDimensions=1  mask(TL_Outport){data={'output',{'name','$B','max',255,'min',0,'class','FCN_REF_ARG','type','UInt8'},'autosar',{'useautosarcommunication',1,'kind',5,'operationargument','AUTOLIV/GlobalDictionary/ClientServerInterfaces/icsModeManagement/Operations/CheckModeStatus/OperationArguments/bModeStatus'},'date',736463.48781274306}}
      settings: CopyFcn=if exist('tl_reset_reviewflag','file')==2,tl_reset_reviewflag(gcbh);end  DeleteFcn=if exist('delete_tlblock','file')==2,delete_tlblock(gcbh);end  NameChangeFcn=if exist('rename_tlblock','file')==2,rename_tlblock(gcbh);end  OpenFcn=if exist('tl_open_blockdlg','file')==2,tl_open_blockdlg(gcbh);else,open_system(gcbh,'parameter');end
      mask Help: eval(['if exist(''tl_online_help'',''file'') == 2, tl_online_help(''Topic'',''TL_Outport''),else, web([''jar:file:///'',matlabroot,''/help/toolbox/simulink/help.jar!/slref/' lower(get_param(gcbh,'Blocktype')) '.html''], ''-helpbrowser''),end'])
      mask Display: plot([0.2 0.35 NaN 0.65 0.8],[0 1 NaN 0 1]);
  wires:
  If Action Subsystem1/1(Out1) -> Merge/1
  Merge/1 -> b8SystemContext/1
  Constant4/1 -> bNoInbibSystemCtxt/2
  bNoInbibSystemCtxt/1 -> If/1
  u16SystemContextsToCheck/1 -> bNoInbibSystemCtxt/1
  If/1 -> If Action Subsystem1/Action
  If/2 -> If Action Subsystem2/Action
  If Action Subsystem2/1(Out1) -> Merge/2

== system PRO_TestHarness/PRO_AC_ProductionCycles/Subsystem/PRO_AC_ProductionCycles/PRO_AC_ProductionCycles/PRO_runProductionCycles/SCA_runCheckSystemContext2 ==
  u16SystemContextsToCheck : Inport  PortDimensions=1  mask(TL_Inport){data={'output',{'class','FCN_ARG','type','UInt16'},'autosar',{'useautosarcommunication',1,'kind',5,'operationargument','AUTOLIV/GlobalDictionary/ClientServerInterfaces/icsModeManagement/Operations/CheckModeStatus/OperationArguments/u32ModesToCheck'},'date',736463.48798901623}}
      settings: CopyFcn=if exist('tl_reset_reviewflag','file')==2,tl_reset_reviewflag(gcbh);end  DeleteFcn=if exist('delete_tlblock','file')==2,delete_tlblock(gcbh);end  NameChangeFcn=if exist('rename_tlblock','file')==2,rename_tlblock(gcbh);end  OpenFcn=if exist('tl_open_blockdlg','file')==2,tl_open_blockdlg(gcbh);else,open_system(gcbh,'parameter');end
      mask Help: eval(['if exist(''tl_online_help'',''file'') == 2, tl_online_help(''Topic'',''TL_Inport''),else, web([''jar:file:///'',matlabroot,''/help/toolbox/simulink/help.jar!/slref/' lower(get_param(gcbh,'Blocktype')) '.html''], ''-helpbrowser''),end'])
      mask Display: plot([0.2 0.35 NaN 0.65 0.8],[0 1 NaN 0 1]);
  Constant4 : Constant  Value=ddv('BFD/CFG_K_MASK_PRO_DTC_INHIBITION_CONTEXT')  OutDataTypeStr=uint8  mask(TL_Constant){data={'output',{'variable','BFD/CFG_K_MASK_PRO_DTC_INHIBITION_CONTEXT'},'date',735893.5675434143}}
      settings: DeleteFcn=if exist('delete_tlblock','file')==2,delete_tlblock(gcbh);end  NameChangeFcn=if exist('rename_tlblock','file')==2,rename_tlblock(gcbh);end  OpenFcn=if exist('tl_open_blockdlg','file')==2,tl_open_blockdlg(gcbh);else,open_system(gcbh,'parameter');end
      mask Help: eval(['if exist(''tl_online_help'',''file'') == 2, tl_online_help(''Topic'',''TL_Constant''),else, web([''jar:file:///'',matlabroot,''/help/toolbox/simulink/help.jar!/slref/' lower(get_param(gcbh,'Blocktype')) '.html''], ''-helpbrowser''),end'])
      mask Display: plot([-0.05, 1.05, NaN, -0.05, 1.05],[.01, .01, NaN, .99, .99])
  Function : tllib/Function  RequirementInfo={} %GIDa_b1474bb6_187e_466c_999e_581558108bd9  data={'stepfunctionname','Rte_Call_pclSystemContext_CheckSystemContext','stepfunctionclass','EXTERN_FCN_SCA','forcereuse',1,'functionarglist',{'u16SystemContextsToCheck';'b8SystemContextStatus_DTCInhibition'},'autosar',{'useautosarspecification',1,'functionrole',3,'clientport','pclModeManagement','operation','CheckModeStatus','isimplementationforsilpil',0,'clientsoftwarecomponent','AUTOLIV/SoftwareComponents/PRO/PRO_AC_ProductionCycles'},'date',736811.3266093171}  displayString=|
      | OPERATION CALL
      | (SYNCHRONOUS)
  If : If  IfExpression=u1
  If Action Subsystem1 : Subsystem  TreatAsAtomicUnit=on
  If Action Subsystem2 : Subsystem  TreatAsAtomicUnit=on
  Merge : Merge  InitialOutput=170  mask(TL_Merge){data={'date',735664.45352688653}}
      settings: CopyFcn=if exist('tl_reset_reviewflag') == 2, tl_reset_reviewflag(gcbh); end  DeleteFcn=if exist('delete_tlblock','file')==2,delete_tlblock(gcbh);end  NameChangeFcn=if exist('rename_tlblock','file')==2,rename_tlblock(gcbh);end  OpenFcn=if exist('tl_open_blockdlg','file')==2,tl_open_blockdlg(gcbh);else,open_system(gcbh,'parameter');end
      mask Help: eval(['if exist(''tl_online_help'',''file'') == 2, tl_online_help(''Topic'',''TL_Merge''),else, web([''jar:file:///'',matlabroot,''/help/toolbox/simulink/help.jar!/slref/' lower(get_param(gcbh,'Blocktype')) '.html''], ''-helpbrowser''),end'])
      mask Display: plot([-0.05, 1.05, NaN, -0.05, 1.05],[.01, .01, NaN, .99, .99])
  bNoInbibSystemCtxt : RelationalOperator  Operator===  OutDataTypeStr=boolean  mask(TL_RelationalOperator){data={'output',{'name','$B'},'date',735419.63408075226}}
      settings: DeleteFcn=if exist('delete_tlblock','file')==2,delete_tlblock(gcbh);end  NameChangeFcn=if exist('rename_tlblock','file')==2,rename_tlblock(gcbh);end  OpenFcn=if exist('tl_open_blockdlg','file')==2,tl_open_blockdlg(gcbh);else,open_system(gcbh,'parameter');end
      mask Help: eval(['if exist(''tl_online_help'',''file'') == 2, tl_online_help(''Topic'',''TL_RelationalOperator''),else, web([''jar:file:///'',matlabroot,''/help/toolbox/simulink/help.jar!/slref/' lower(get_param(gcbh,'Blocktype')) '.html''], ''-helpbrowser''),end'])
      mask Display: plot([-0.05, 1.05, NaN, -0.05, 1.05],[.01, .01, NaN, .99, .99])
  b8SystemContext : Outport  RequirementInfo={} %GIDa_bb9c4d9c_1187_4785_b94a_2ddaf6c00cf9  PortDimensions=1  mask(TL_Outport){data={'output',{'name','$B','max',255,'min',0,'class','FCN_REF_ARG','type','UInt8'},'autosar',{'useautosarcommunication',1,'kind',5,'operationargument','AUTOLIV/GlobalDictionary/ClientServerInterfaces/icsModeManagement/Operations/CheckModeStatus/OperationArguments/bModeStatus'},'date',736463.48816747684}}
      settings: CopyFcn=if exist('tl_reset_reviewflag','file')==2,tl_reset_reviewflag(gcbh);end  DeleteFcn=if exist('delete_tlblock','file')==2,delete_tlblock(gcbh);end  NameChangeFcn=if exist('rename_tlblock','file')==2,rename_tlblock(gcbh);end  OpenFcn=if exist('tl_open_blockdlg','file')==2,tl_open_blockdlg(gcbh);else,open_system(gcbh,'parameter');end
      mask Help: eval(['if exist(''tl_online_help'',''file'') == 2, tl_online_help(''Topic'',''TL_Outport''),else, web([''jar:file:///'',matlabroot,''/help/toolbox/simulink/help.jar!/slref/' lower(get_param(gcbh,'Blocktype')) '.html''], ''-helpbrowser''),end'])
      mask Display: plot([0.2 0.35 NaN 0.65 0.8],[0 1 NaN 0 1]);
  wires:
  If Action Subsystem1/1(Out1) -> Merge/1
  Merge/1 -> b8SystemContext/1
  Constant4/1 -> bNoInbibSystemCtxt/2
  bNoInbibSystemCtxt/1 -> If/1
  u16SystemContextsToCheck/1 -> bNoInbibSystemCtxt/1
  If/1 -> If Action Subsystem1/Action
  If/2 -> If Action Subsystem2/Action
  If Action Subsystem2/1(Out1) -> Merge/2
